simulink model "HybridControllerD3D3_Vconst"  (Simulink 7.9)
settings: Solver=FixedStepDiscrete  StartTime=0.0  StopTime=inf  RelTol=1e-3
PreLoadFcn:
  | initializeSimulation
values from neighbouring files (symbols this model uses):
  nAct = 8    [initializeSimulation.m]
  nDOF = 2    [initializeSimulation.m]
  nDout = 4    [initializeSimulation.m]
  node = completenodestruct(node)    [initializeSimulation.m]
undefined symbols (not defined in the file or in its folder): dofID, HybridCtrlParameters, vDOF, vDOFmax
libraries: xpclib x10, xpcsystranlib x4, simulink x4
CloseFcn:
  | rtwprivate ssgencode ModelCloseRequest scrnet_receiver
settings Model: Creator=Andreas Schellenberg  LastModifiedBy=Andreas  ExtModeArmWhenConnect=off  BufferReuse=off
settings DataIOCC: LimitDataPoints=off  SaveOutput=off  SignalLogging=off  SaveTime=off  SignalLoggingName=sigsOut
settings OptimizationCC: BlockReduction=off  OptimizeBlockIOStorage=off  BufferReuse=off  ExpressionFolding=off  FoldNonRolledExpr=off  LocalBlockOutputs=off  StateBitsets=on  DataBitsets=on  InitFltsAndDblsToZero=on  EfficientFloat2IntCast=on  SimCompilerOptimization=On
settings DebuggingCC: SaveWithParameterizedLinksMsg=none  CheckSSInitialOutputMsg=off  SolverPrmCheckMsg=none  FcnCallInpInsideContextMsg=Use local settings  StrictBusMsg=None
settings HardwareCC: ProdIntDivRoundTo=Zero  ProdEndianess=LittleEndian  ProdHWDeviceType=Generic->32-bit x86 compatible  TargetIntDivRoundTo=Zero  TargetEndianess=LittleEndian  TargetHWDeviceType=Intel->x86/Pentium
settings SFSimCC: SimCustomHeaderCode="#include \"PredictorCorrector.h\""  SimUserSources=PredictorCorrector.c  SimUserIncludeDirs=D:\PredictorCorrector\HybridSimToolbox  SimParseCustomCode=off
settings RTWCC: SystemTargetFile=xpctarget.tlc  TemplateMakefile=xpc_default_tmf  Description=xPC Target  ProcessScript=xpctarget_make_rtw_hook  CustomHeaderCode="#include \"PredictorCorrector.h\""  CustomInclude=D:\PredictorCorrector\HybridSimToolbox  CustomSource=PredictorCorrector.c  IncludeERTFirstTime=on  RTWCompilerOptimization=On
settings xpcTargetCC: TargetFcnLib=ansi_tfl_tmw.mat  CodeReplacementLibrary=XPC_BLAS  CodeExecutionProfiling=off  ParMdlRefBuildCompliant=on  ConcurrentExecutionCompliant=on  CombineSignalStateStructs=off  PortableWordSizes=off  GRTInterface=on  xPCTaskExecutionProfile=off  xPCRL32EventNumber=5000  RL32IRQSourceModifier=11  xPCIRQSourceBoard=Scramnet_SC150+  xPCLoadParamSetFile=off  xPCConcurrentTasks=off  xPCEnableSFAnimation=off

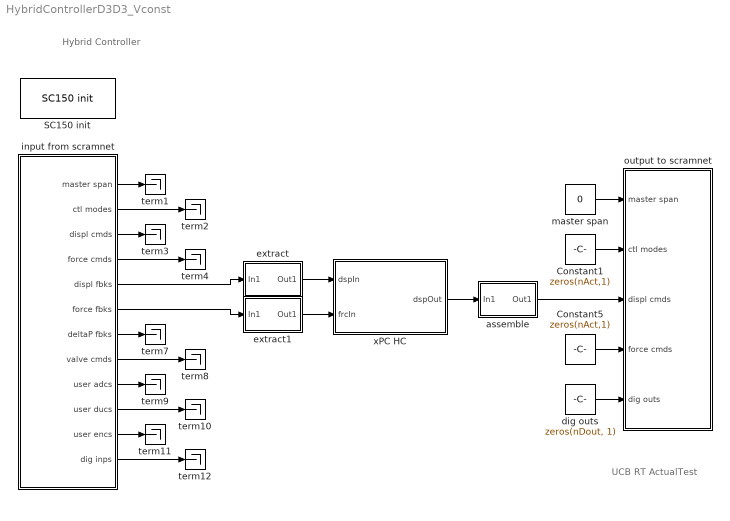
== system HybridControllerD3D3_Vconst ==
  note: Hybrid Controller
  note: UCB RT ActualTest
  Constant1 : Constant  Value=zeros(nAct,1)
  Constant5 : Constant  Value=zeros(nAct,1)
  SC150 init : xpcsystranlib/Shared Memory/SC150 init   node=node  pci=-1
  assemble : Subsystem  mask(to Actuators){id=[2 3], size=nAct}
      mask prompts: id "Index Vector: id"; size "Vector Size: size"
      mask help: To select to which actuator(s) the signals are going to
      mask Display: disp('Assemble')
  dig outs : Constant  Value=zeros(nDout, 1)  OutDataTypeStr=uint32
  extract : Subsystem  mask(from Actuators){id=[2 3], size=nAct}
      mask prompts: id "Index Vector: id"; size "Vector Size: size"
      mask help: To select from which actuator(s) the signals are coming from
      mask Display: disp('Extract')
  extract1 : Subsystem  mask(from Actuators){id=[2 3], size=nAct}
      mask prompts: id "Index Vector: id"; size "Vector Size: size"
      mask help: To select from which actuator(s) the signals are coming from
      mask Display: disp('Extract')
  input from scramnet : Subsystem
  master span : Constant  Value=0
  output to scramnet : Subsystem
  term{1..4,7..12} (10 alike) : Terminator
  xPC HC : Subsystem  mask(Hybrid Controller: D3/D3){nDOF=nDOF, dtInt=HybridCtrlParameters.dtInt, dtSim=HybridCtrlParameters.dtSim, dtCon=HybridCtrlParameters.dtCon, N=HybridCtrlParameters.N, iDelay=HybridCtrlParameters.iDelay}
      mask prompts: nDOF "Number of DOF: nDOF"; dtInt "Integration time step: dtInt"; dtSim "Simulation time step: dtSim"; dtCon "Controller time step: dtCon"; N "Maximum number of substeps: N"; iDelay "Number of delay steps: iDelay"
      mask help: Hybrid Controller using C0-continuous cubic Lagrange interpolation for prediction and correction
      mask Display: disp('xPC Target\nHybrid Controller\n(D3/D3 Vconst)')
  wires:
  input from scramnet/10(user ducs) -> term10/1
  input from scramnet/12(dig inps) -> term12/1
  input from scramnet/2(ctl modes) -> term2/1
  input from scramnet/4(force cmds) -> term4/1
  input from scramnet/8(valve cmds) -> term8/1
  input from scramnet/1(master span) -> term1/1
  input from scramnet/7(deltaP fbks) -> term7/1
  input from scramnet/9(user adcs) -> term9/1
  input from scramnet/11(user encs) -> term11/1
  master span/1 -> output to scramnet/1(master span)
  Constant5/1 -> output to scramnet/4(force cmds)
  Constant1/1 -> output to scramnet/2(ctl modes)
  input from scramnet/3(displ cmds) -> term3/1
  input from scramnet/5(displ fbks) -> extract/1(In1)
  dig outs/1 -> output to scramnet/5(dig outs)
  extract/1(Out1) -> xPC HC/1(dspIn)
  xPC HC/1(dspOut) -> assemble/1(In1)
  assemble/1(Out1) -> output to scramnet/3(displ cmds)
  input from scramnet/6(force fbks) -> extract1/1(In1)
  extract1/1(Out1) -> xPC HC/2(frcIn)

== system HybridControllerD3D3_Vconst/assemble ==
  In1 : Inport
  Assignment : Assignment  OutputInitialize=Specify size for each dimension in table  IndexOptions=Index vector (port)  Indices=1  OutputSizes=size
  Constant : Constant  Value=id
  Out1 : Outport
  wires:
  Constant/1 -> Assignment/2
  Assignment/1 -> Out1/1
  In1/1 -> Assignment/1

== system HybridControllerD3D3_Vconst/extract ==
  In1 : Inport
  Selector : Selector  InputPortWidth=size  IndexOptions=Index vector (dialog)  Indices=id  OutputSizes=1
  Out1 : Outport
  wires:
  Selector/1 -> Out1/1
  In1/1 -> Selector/1

== system HybridControllerD3D3_Vconst/extract1 ==
  In1 : Inport
  Selector : Selector  InputPortWidth=size  IndexOptions=Index vector (dialog)  Indices=id  OutputSizes=1
  Out1 : Outport
  wires:
  Selector/1 -> Out1/1
  In1/1 -> Selector/1

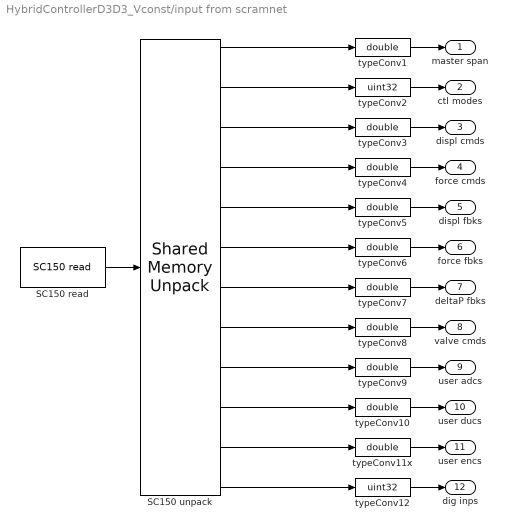
== system HybridControllerD3D3_Vconst/input from scramnet ==
  SC150 read : xpcsystranlib/Shared Memory/SC150 read   partition=node.Partitions(12:23)  errorport=off  ts=samplePeriod  pci=-1
  SC150 unpack : xpclib/Shared Memory/Shared Memory Unpack   partition=node.Partitions(12:23)
  typeConv{1,3..10} (9 alike) : DataTypeConversion  OutDataTypeStr=double  SaturateOnIntegerOverflow=on  RndMeth=Zero
  typeConv11x : DataTypeConversion  OutDataTypeStr=double  SaturateOnIntegerOverflow=on  RndMeth=Zero
  typeConv12 : DataTypeConversion  OutDataTypeStr=uint32  SaturateOnIntegerOverflow=on  RndMeth=Zero
  typeConv2 : DataTypeConversion  OutDataTypeStr=uint32  SaturateOnIntegerOverflow=on  RndMeth=Zero
  master span : Outport
  ctl modes : Outport  Port=2
  displ cmds : Outport  Port=3
  force cmds : Outport  Port=4
  displ fbks : Outport  Port=5
  force fbks : Outport  Port=6
  deltaP fbks : Outport  Port=7
  valve cmds : Outport  Port=8
  user adcs : Outport  Port=9
  user ducs : Outport  Port=10
  user encs : Outport  Port=11
  dig inps : Outport  Port=12
  wires:
  typeConv11x/1 -> user encs/1
  typeConv10/1 -> user ducs/1
  typeConv12/1 -> dig inps/1
  typeConv9/1 -> user adcs/1
  typeConv8/1 -> valve cmds/1
  typeConv7/1 -> deltaP fbks/1
  typeConv6/1 -> force fbks/1
  typeConv5/1 -> displ fbks/1
  typeConv4/1 -> force cmds/1
  typeConv3/1 -> displ cmds/1
  typeConv1/1 -> master span/1
  SC150 read/1 -> SC150 unpack/1
  typeConv2/1 -> ctl modes/1
  SC150 unpack/1 -> typeConv1/1
  SC150 unpack/2 -> typeConv2/1
  SC150 unpack/3 -> typeConv3/1
  SC150 unpack/4 -> typeConv4/1
  SC150 unpack/5 -> typeConv5/1
  SC150 unpack/6 -> typeConv6/1
  SC150 unpack/7 -> typeConv7/1
  SC150 unpack/8 -> typeConv8/1
  SC150 unpack/9 -> typeConv9/1
  SC150 unpack/10 -> typeConv10/1
  SC150 unpack/11 -> typeConv11x/1
  SC150 unpack/12 -> typeConv12/1

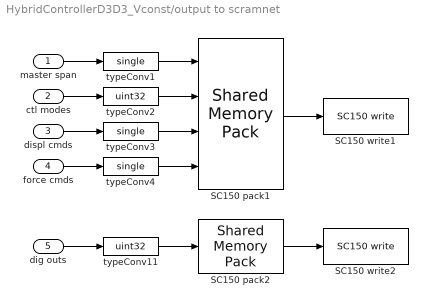
== system HybridControllerD3D3_Vconst/output to scramnet ==
  master span : Inport
  ctl modes : Inport  Port=2
  displ cmds : Inport  Port=3
  force cmds : Inport  Port=4
  dig outs : Inport  Port=5
  SC150 pack1 : xpclib/Shared Memory/Shared Memory Pack   partition=node.Partitions(1:4)
  SC150 pack2 : xpclib/Shared Memory/Shared Memory Pack   partition=node.Partitions(11)
  SC150 write1 : xpcsystranlib/Shared Memory/SC150 write   partition=node.Partitions(1:4)  errorport=off  ts=samplePeriod  pci=-1
  SC150 write2 : xpcsystranlib/Shared Memory/SC150 write   partition=node.Partitions(11)  errorport=off  ts=samplePeriod  pci=-1
  typeConv1 : DataTypeConversion  OutDataTypeStr=single  SaturateOnIntegerOverflow=on  RndMeth=Zero
  typeConv11 : DataTypeConversion  OutDataTypeStr=uint32  SaturateOnIntegerOverflow=on  RndMeth=Zero
  typeConv2 : DataTypeConversion  OutDataTypeStr=uint32  SaturateOnIntegerOverflow=on  RndMeth=Zero
  typeConv3 : DataTypeConversion  OutDataTypeStr=single  SaturateOnIntegerOverflow=on  RndMeth=Zero
  typeConv4 : DataTypeConversion  OutDataTypeStr=single  SaturateOnIntegerOverflow=on  RndMeth=Zero
  wires:
  dig outs/1 -> typeConv11/1
  force cmds/1 -> typeConv4/1
  master span/1 -> typeConv1/1
  SC150 pack1/1 -> SC150 write1/1
  displ cmds/1 -> typeConv3/1
  ctl modes/1 -> typeConv2/1
  typeConv1/1 -> SC150 pack1/1
  typeConv2/1 -> SC150 pack1/2
  typeConv3/1 -> SC150 pack1/3
  typeConv4/1 -> SC150 pack1/4
  SC150 pack2/1 -> SC150 write2/1
  typeConv11/1 -> SC150 pack2/1

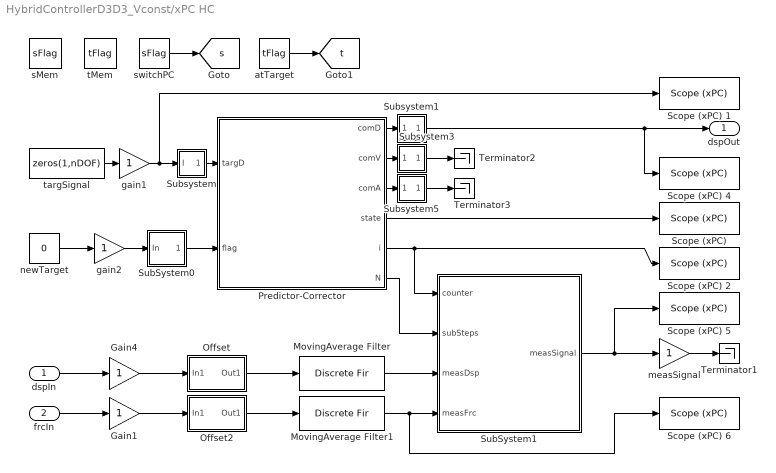
== system HybridControllerD3D3_Vconst/xPC HC ==
  dspIn : Inport
  frcIn : Inport  Port=2
  Gain1 : Gain  SaturateOnIntegerOverflow=on  OutDataTypeStr=Inherit: Same as input  ParamDataTypeStr=Inherit: Same as input
  Gain4 : Gain  SaturateOnIntegerOverflow=on  OutDataTypeStr=Inherit: Same as input  ParamDataTypeStr=Inherit: Same as input
  MovingAverage Filter : DiscreteFir  Coefficients=1/numSample*ones(1,numSample)  mask(Moving Average Filter){numSample=1}
      mask prompts: numSample "Number of Samples: numSample"
      mask help:
      | Moving average filter by using discrete FIR filter.
      | Set numSample = 1 for no filtering.
      mask Display: fprintf('MovingAverage\nFilter')
  MovingAverage Filter1 : DiscreteFir  Coefficients=1/numSample*ones(1,numSample)  mask(Moving Average Filter){numSample=1}
      mask prompts: numSample "Number of Samples: numSample"
      mask help:
      | Moving average filter by using discrete FIR filter.
      | Set numSample = 1 for no filtering.
      mask Display: fprintf('MovingAverage\nFilter')
  Offset : Subsystem  mask(Signal Offset){nS=nDOF, nOffset=-1, dt=dtCon}
      mask prompts: nS "Number of Signals: nS"; nOffset "Number of samples to initialize offset: nOffset"; dt "Sample time: dt"
      mask help:
      | Offset signal by average of signal over initial number of samples.
      | Set nOffset = -1 for no signal offset.
      mask Display: fprintf('Signal\nOffset')
  Offset2 : Subsystem  mask(Signal Offset){nS=nDOF, nOffset=-1, dt=dtCon}
      mask prompts: nS "Number of Signals: nS"; nOffset "Number of samples to initialize offset: nOffset"; dt "Sample time: dt"
      mask help:
      | Offset signal by average of signal over initial number of samples.
      | Set nOffset = -1 for no signal offset.
      mask Display: fprintf('Signal\nOffset')
  Predictor-Corrector : Stateflow chart  TreatAsAtomicUnit=on
  "Scope (xPC) " : xpclib/Misc./Scope (xPC)   scopeno=8  scopetype=File  autostart=on  viewmode=Graphical redraw  formatstr='%15.6f'  grid=on  ylimits=[0,3]  nosamples=4096  noprepostsamples=0  interleave=1  triggermode=FreeRun  triggersignal=1  triggerlevel=0.0  triggerslope=Either  triggerscope=1  triggersample=0  filename=state1.dat  mode=Lazy  writesize=512  autorestart=on  dynamicfilemode=off  maxwritefilesize=512*1024^2
  Scope (xPC) 1 : xpclib/Misc./Scope (xPC)   scopeno=4  scopetype=File  autostart=on  viewmode=Numerical  formatstr='%15.6f'  grid=on  ylimits=[-4,4]  nosamples=4096  noprepostsamples=0  interleave=1  triggermode=FreeRun  triggersignal=1  triggerlevel=0.0  triggerslope=Either  triggerscope=1  triggersample=0  filename=targDsp1.dat  mode=Lazy  writesize=512  autorestart=on  dynamicfilemode=off  maxwritefilesize=512*1024^2
  Scope (xPC) 2 : xpclib/Misc./Scope (xPC)   scopeno=1  scopetype=File  autostart=on  viewmode=Numerical  formatstr='%15.6f'  grid=on  ylimits=[0,3]  nosamples=4096  noprepostsamples=0  interleave=1  triggermode=FreeRun  triggersignal=1  triggerlevel=0.0  triggerslope=Either  triggerscope=1  triggersample=0  filename=count1.dat  mode=Lazy  writesize=512  autorestart=on  dynamicfilemode=off  maxwritefilesize=512*1024^2
  Scope (xPC) 4 : xpclib/Misc./Scope (xPC)   scopeno=5  scopetype=File  autostart=on  viewmode=Numerical  formatstr='%15.6f'  grid=on  ylimits=[-4,4]  nosamples=4096  noprepostsamples=0  interleave=1  triggermode=FreeRun  triggersignal=1  triggerlevel=0.0  triggerslope=Either  triggerscope=1  triggersample=0  filename=commDsp1.dat  mode=Lazy  writesize=512  autorestart=on  dynamicfilemode=off  maxwritefilesize=512*1024^2
  Scope (xPC) 5 : xpclib/Misc./Scope (xPC)   scopeno=2  scopetype=File  autostart=on  viewmode=Numerical  formatstr='%15.6f'  grid=on  ylimits=[-4,4]  nosamples=4096  noprepostsamples=0  interleave=1  triggermode=FreeRun  triggersignal=1  triggerlevel=0.0  triggerslope=Either  triggerscope=1  triggersample=0  filename=measDsp1.dat  mode=Lazy  writesize=512  autorestart=on  dynamicfilemode=off  maxwritefilesize=512*1024^2
  Scope (xPC) 6 : xpclib/Misc./Scope (xPC)   scopeno=3  scopetype=File  autostart=on  viewmode=Numerical  formatstr='%15.6f'  grid=on  ylimits=[0,3]  nosamples=4096  noprepostsamples=0  interleave=1  triggermode=FreeRun  triggersignal=1  triggerlevel=0.0  triggerslope=Either  triggerscope=1  triggersample=0  filename=measFrc1.dat  mode=Lazy  writesize=512  autorestart=on  dynamicfilemode=off  maxwritefilesize=512*1024^2
  SubSystem0 : Subsystem
  SubSystem1 : Subsystem
  Subsystem : Subsystem
      mask Display: disp('I/O')
  Subsystem1 : Subsystem
      mask Display: disp('I/O')
  Subsystem3 : Subsystem
      mask Display: disp('I/O')
  Subsystem5 : Subsystem
      mask Display: disp('I/O')
  Terminator1 : Terminator
  Terminator2 : Terminator
  Terminator3 : Terminator
  atTarget : DataStoreRead  DataStoreName=tFlag  SampleTime=dtCon
  gain1 : Gain
  gain2 : Gain
  measSignal : Gain
  newTarget : Constant  Value=0  SampleTime=dtCon
  sMem : DataStoreMemory  DataStoreName=sFlag  OutDataTypeStr=double
  switchPC : DataStoreRead  DataStoreName=sFlag  SampleTime=dtCon
  tMem : DataStoreMemory  DataStoreName=tFlag  OutDataTypeStr=double
  targSignal : Constant  Value=zeros(1,nDOF)  SampleTime=dtCon
  dspOut : Outport
  tag scope: s=global, t=global
  wires:
  frcIn/1 -> Gain1/1
  measSignal/1 -> Terminator1/1
  dspIn/1 -> Gain4/1
  SubSystem1/1(measSignal) -> measSignal/1, Scope (xPC) 5/1
  Predictor-Corrector/5(i) -> Scope (xPC) 2/1, SubSystem1/1(counter)
  Predictor-Corrector/4(state) -> "Scope (xPC) "/1
  Offset/1(Out1) -> MovingAverage Filter/1
  SubSystem0/1(Out) -> Predictor-Corrector/2(flag)
  newTarget/1 -> gain2/1
  gain2/1 -> SubSystem0/1(In)
  switchPC/1 -> [s]
  atTarget/1 -> [t]
  targSignal/1 -> gain1/1
  gain1/1 -> Scope (xPC) 1/1, Subsystem/1(I)
  Subsystem1/1(Out) -> dspOut/1, Scope (xPC) 4/1
  Subsystem/1(O) -> Predictor-Corrector/1(targD)
  MovingAverage Filter/1 -> SubSystem1/3(measDsp)
  MovingAverage Filter1/1 -> Scope (xPC) 6/1, SubSystem1/4(measFrc)
  Predictor-Corrector/1(comD) -> Subsystem1/1(In)
  Predictor-Corrector/2(comV) -> Subsystem3/1(In)
  Predictor-Corrector/3(comA) -> Subsystem5/1(In)
  Subsystem3/1(Out) -> Terminator2/1
  Subsystem5/1(Out) -> Terminator3/1
  Gain4/1 -> Offset/1(In1)
  Gain1/1 -> Offset2/1(In1)
  Offset2/1(Out1) -> MovingAverage Filter1/1
  Predictor-Corrector/6(N) -> SubSystem1/2(subSteps)

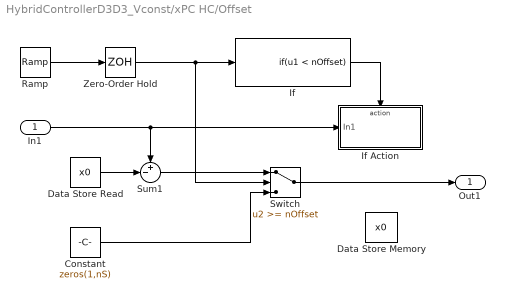
== system HybridControllerD3D3_Vconst/xPC HC/Offset ==
  In1 : Inport
  Constant : Constant  Value=zeros(1,nS)
  Data Store Memory : DataStoreMemory  DataStoreName=x0  InitialValue=zeros(1,nS)  OutDataTypeStr=double
  Data Store Read : DataStoreRead  DataStoreName=x0  SampleTime=dt
  If : If  IfExpression=u1 < nOffset  ShowElse=off
  If Action : Subsystem  TreatAsAtomicUnit=on
  Ramp : simulink/Sources/Ramp  slope=1/dt  start=0  X0=0
  Sum1 : Sum  Inputs=+-|  SaturateOnIntegerOverflow=on  InputSameDT=on  OutDataTypeStr=Inherit: Same as first input
  Switch : Switch  Threshold=nOffset  SaturateOnIntegerOverflow=on  InputSameDT=on
  Zero-Order Hold : ZeroOrderHold  SampleTime=dt
  Out1 : Outport
  wires:
  Switch/1 -> Out1/1
  Sum1/1 -> Switch/1
  Data Store Read/1 -> Sum1/2
  In1/1 -> If Action/1(In1), Sum1/1
  Constant/1 -> Switch/3
  Zero-Order Hold/1 -> Switch/2, If/1
  If/1 -> If Action/Action
  Ramp/1 -> Zero-Order Hold/1

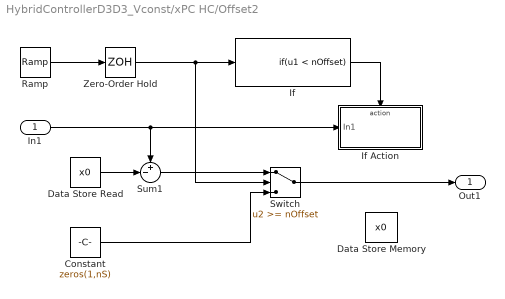
== system HybridControllerD3D3_Vconst/xPC HC/Offset2 ==
  In1 : Inport
  Constant : Constant  Value=zeros(1,nS)
  Data Store Memory : DataStoreMemory  DataStoreName=x0  InitialValue=zeros(1,nS)  OutDataTypeStr=double
  Data Store Read : DataStoreRead  DataStoreName=x0  SampleTime=dt
  If : If  IfExpression=u1 < nOffset  ShowElse=off
  If Action : Subsystem  TreatAsAtomicUnit=on
  Ramp : simulink/Sources/Ramp  slope=1/dt  start=0  X0=0
  Sum1 : Sum  Inputs=+-|  SaturateOnIntegerOverflow=on  InputSameDT=on  OutDataTypeStr=Inherit: Same as first input
  Switch : Switch  Threshold=nOffset  SaturateOnIntegerOverflow=on  InputSameDT=on
  Zero-Order Hold : ZeroOrderHold  SampleTime=dt
  Out1 : Outport
  wires:
  Ramp/1 -> Zero-Order Hold/1
  If/1 -> If Action/Action
  Zero-Order Hold/1 -> If/1, Switch/2
  Constant/1 -> Switch/3
  In1/1 -> Sum1/1, If Action/1(In1)
  Data Store Read/1 -> Sum1/2
  Sum1/1 -> Switch/1
  Switch/1 -> Out1/1

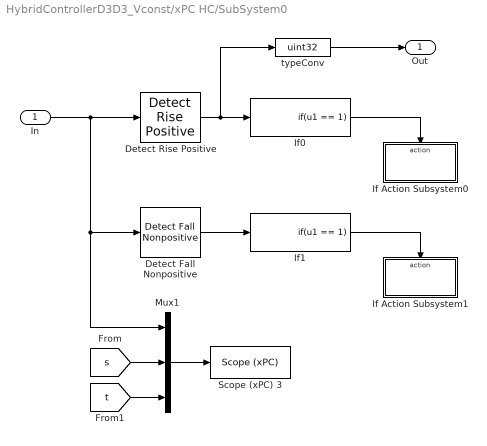
== system HybridControllerD3D3_Vconst/xPC HC/SubSystem0 ==
  In : Inport
  Detect Fall Nonpositive : simulink/Logic and Bit Operations/Detect Fall Nonpositive  vinit=0  InputProcessing=Inherited  OutDataTypeStr=uint8
  Detect Rise Positive : simulink/Logic and Bit Operations/Detect Rise Positive  vinit=0  InputProcessing=Inherited  OutDataTypeStr=uint8
  If Action Subsystem0 : Subsystem  TreatAsAtomicUnit=on
  If Action Subsystem1 : Subsystem  TreatAsAtomicUnit=on
  If0 : If  IfExpression=u1 == 1  ShowElse=off
  If1 : If  IfExpression=u1 == 1  ShowElse=off
  Mux1 : Mux  Inputs=3
  Scope (xPC) 3 : xpclib/Misc./Scope (xPC)   scopeno=6  scopetype=File  autostart=on  viewmode=Numerical  formatstr='%15.6f'  grid=on  ylimits=[0,3]  nosamples=4096  noprepostsamples=0  interleave=1  triggermode=FreeRun  triggersignal=1  triggerlevel=0.0  triggerslope=Either  triggerscope=1  triggersample=0  filename=flag1.dat  mode=Lazy  writesize=512  autorestart=on  dynamicfilemode=off  maxwritefilesize=512*1024^2
  typeConv : DataTypeConversion  OutDataTypeStr=uint32  SaturateOnIntegerOverflow=on  RndMeth=Zero
  Out : Outport
  wires:
  In/1 -> Detect Rise Positive/1, Detect Fall Nonpositive/1, Mux1/1
  Detect Rise Positive/1 -> If0/1, typeConv/1
  Detect Fall Nonpositive/1 -> If1/1
  If1/1 -> If Action Subsystem1/Action
  If0/1 -> If Action Subsystem0/Action
  typeConv/1 -> Out/1
  Mux1/1 -> Scope (xPC) 3/1
  [s] -> Mux1/2
  [t] -> Mux1/3

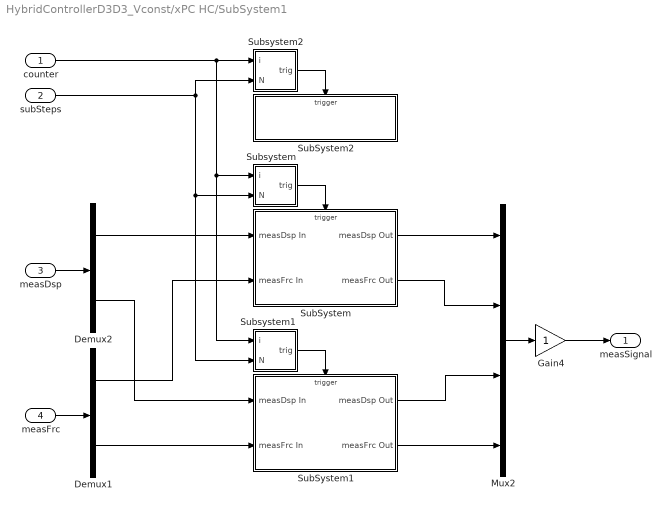
== system HybridControllerD3D3_Vconst/xPC HC/SubSystem1 ==
  counter : Inport
  subSteps : Inport  Port=2
  measDsp : Inport  Port=3
  measFrc : Inport  Port=4
  Demux1 : Demux  Outputs=2
  Demux2 : Demux  Outputs=2
  Gain4 : Gain  SaturateOnIntegerOverflow=on  OutDataTypeStr=Inherit: Same as input  ParamDataTypeStr=Inherit: Same as input
  Mux2 : Mux
  SubSystem : Subsystem  TreatAsAtomicUnit=on
  SubSystem1 : Subsystem  TreatAsAtomicUnit=on
  SubSystem2 : Subsystem  TreatAsAtomicUnit=on
  Subsystem : Subsystem
  Subsystem1 : Subsystem
  Subsystem2 : Subsystem
  measSignal : Outport
  wires:
  Subsystem/1(trig) -> SubSystem/Trigger
  Subsystem1/1(trig) -> SubSystem1/Trigger
  Subsystem2/1(trig) -> SubSystem2/Trigger
  Mux2/1 -> Gain4/1
  SubSystem/1(measDsp Out) -> Mux2/1
  counter/1 -> Subsystem/1(i), Subsystem1/1(i), Subsystem2/1(i)
  Gain4/1 -> measSignal/1
  SubSystem/2(measFrc Out) -> Mux2/2
  SubSystem1/1(measDsp Out) -> Mux2/3
  SubSystem1/2(measFrc Out) -> Mux2/4
  measDsp/1 -> Demux2/1
  measFrc/1 -> Demux1/1
  Demux2/1 -> SubSystem/1(measDsp In)
  Demux2/2 -> SubSystem1/1(measDsp In)
  Demux1/1 -> SubSystem/2(measFrc In)
  Demux1/2 -> SubSystem1/2(measFrc In)
  subSteps/1 -> Subsystem2/2(N), Subsystem/2(N), Subsystem1/2(N)

== system HybridControllerD3D3_Vconst/xPC HC/Subsystem ==
  I : Inport  PortDimensions=nAct
  Dummy Aug : Mux  Inputs=[nAct 1]
  Dummy Zero : Constant  Value=0  OutDataTypeStr=double  SampleTime=dtCon
  O : Outport  PortDimensions=nAct+1
  wires:
  Dummy Zero/1 -> Dummy Aug/2
  I/1 -> Dummy Aug/1
  Dummy Aug/1 -> O/1

== system HybridControllerD3D3_Vconst/xPC HC/Subsystem1 ==
  In : Inport  PortDimensions=nAct+1
  Dummy Trn : Demux  Outputs=[nAct 1]
  Terminator3 : Terminator
  Out : Outport  PortDimensions=nAct
  wires:
  Dummy Trn/2 -> Terminator3/1
  Dummy Trn/1 -> Out/1
  In/1 -> Dummy Trn/1

== system HybridControllerD3D3_Vconst/xPC HC/Subsystem3 ==
  In : Inport  PortDimensions=nAct+1
  Dummy Trn : Demux  Outputs=[nAct 1]
  Terminator3 : Terminator
  Out : Outport  PortDimensions=nAct
  wires:
  Dummy Trn/2 -> Terminator3/1
  Dummy Trn/1 -> Out/1
  In/1 -> Dummy Trn/1

== system HybridControllerD3D3_Vconst/xPC HC/Subsystem5 ==
  In : Inport  PortDimensions=nAct+1
  Dummy Trn : Demux  Outputs=[nAct 1]
  Terminator3 : Terminator
  Out : Outport  PortDimensions=nAct
  wires:
  Dummy Trn/2 -> Terminator3/1
  Dummy Trn/1 -> Out/1
  In/1 -> Dummy Trn/1

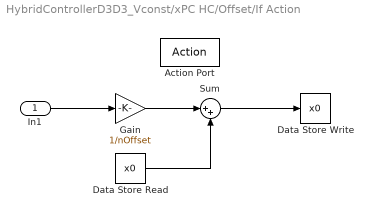
== system HybridControllerD3D3_Vconst/xPC HC/Offset/If Action ==
  In1 : Inport
  Action Port : ActionPort  PropagateVarSize=During execution
  Data Store Read : DataStoreRead  DataStoreName=x0  SampleTime=dt
  Data Store Write : DataStoreWrite  DataStoreName=x0
  Gain : Gain  Gain=1/nOffset  SaturateOnIntegerOverflow=on  OutDataTypeStr=Inherit: Same as input  ParamDataTypeStr=Inherit: Same as input
  Sum : Sum  Inputs=|++  SaturateOnIntegerOverflow=on  InputSameDT=on  OutDataTypeStr=Inherit: Same as first input
  wires:
  Data Store Read/1 -> Sum/2
  Sum/1 -> Data Store Write/1
  Gain/1 -> Sum/1
  In1/1 -> Gain/1

== system HybridControllerD3D3_Vconst/xPC HC/Offset2/If Action ==
  In1 : Inport
  Action Port : ActionPort  PropagateVarSize=During execution
  Data Store Read : DataStoreRead  DataStoreName=x0  SampleTime=dt
  Data Store Write : DataStoreWrite  DataStoreName=x0
  Gain : Gain  Gain=1/nOffset  SaturateOnIntegerOverflow=on  OutDataTypeStr=Inherit: Same as input  ParamDataTypeStr=Inherit: Same as input
  Sum : Sum  Inputs=|++  SaturateOnIntegerOverflow=on  InputSameDT=on  OutDataTypeStr=Inherit: Same as first input
  wires:
  In1/1 -> Gain/1
  Gain/1 -> Sum/1
  Sum/1 -> Data Store Write/1
  Data Store Read/1 -> Sum/2

== system HybridControllerD3D3_Vconst/xPC HC/SubSystem0/If Action Subsystem0 ==
  Action Port : ActionPort  PropagateVarSize=During execution
  Data Store Write0 : DataStoreWrite  DataStoreName=sFlag
  Data Store Write1 : DataStoreWrite  DataStoreName=tFlag
  atTargetFlag : Constant  Value=0  SampleTime=dtCon
  switchFlag : Constant  SampleTime=dtCon
  wires:
  atTargetFlag/1 -> Data Store Write1/1
  switchFlag/1 -> Data Store Write0/1

== system HybridControllerD3D3_Vconst/xPC HC/SubSystem0/If Action Subsystem1 ==
  Action Port : ActionPort  PropagateVarSize=During execution
  Data Store Write0 : DataStoreWrite  DataStoreName=sFlag
  switchFlag : Constant  Value=0  SampleTime=dtCon
  wires:
  switchFlag/1 -> Data Store Write0/1

== system HybridControllerD3D3_Vconst/xPC HC/SubSystem1/SubSystem ==
  measDsp In : Inport
  measFrc In : Inport  Port=2
  Trigger : TriggerPort
  measDsp Out : Outport  InitialOutput=[0]
  measFrc Out : Outport  Port=2  InitialOutput=[0]
  wires:
  measFrc In/1 -> measFrc Out/1
  measDsp In/1 -> measDsp Out/1

== system HybridControllerD3D3_Vconst/xPC HC/SubSystem1/SubSystem1 ==
  measDsp In : Inport
  measFrc In : Inport  Port=2
  Trigger : TriggerPort
  measDsp Out : Outport  InitialOutput=[0]
  measFrc Out : Outport  Port=2  InitialOutput=[0]
  wires:
  measFrc In/1 -> measFrc Out/1
  measDsp In/1 -> measDsp Out/1

== system HybridControllerD3D3_Vconst/xPC HC/SubSystem1/SubSystem2 ==
  Trigger : TriggerPort
  Data Store Write : DataStoreWrite  DataStoreName=tFlag
  atTargetFlag : Constant  OutDataTypeStr=uint32  SampleTime=-1
  wires:
  atTargetFlag/1 -> Data Store Write/1

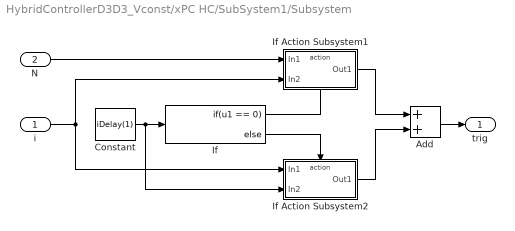
== system HybridControllerD3D3_Vconst/xPC HC/SubSystem1/Subsystem ==
  i : Inport
  N : Inport  Port=2
  Add : Sum
  Constant : Constant  Value=iDelay(1)
  If : If  IfExpression=u1 == 0
  If Action Subsystem1 : Subsystem  TreatAsAtomicUnit=on
  If Action Subsystem2 : Subsystem  TreatAsAtomicUnit=on
  trig : Outport
  wires:
  Constant/1 -> If/1, If Action Subsystem2/2(In2)
  If/1 -> If Action Subsystem1/Action
  If/2 -> If Action Subsystem2/Action
  If Action Subsystem1/1(Out1) -> Add/1
  If Action Subsystem2/1(Out1) -> Add/2
  Add/1 -> trig/1
  i/1 -> If Action Subsystem1/2(In2), If Action Subsystem2/1(In1)
  N/1 -> If Action Subsystem1/1(In1)

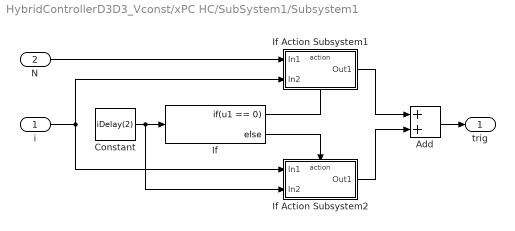
== system HybridControllerD3D3_Vconst/xPC HC/SubSystem1/Subsystem1 ==
  i : Inport
  N : Inport  Port=2
  Add : Sum
  Constant : Constant  Value=iDelay(2)
  If : If  IfExpression=u1 == 0
  If Action Subsystem1 : Subsystem  TreatAsAtomicUnit=on
  If Action Subsystem2 : Subsystem  TreatAsAtomicUnit=on
  trig : Outport
  wires:
  Constant/1 -> If/1, If Action Subsystem2/2(In2)
  If/1 -> If Action Subsystem1/Action
  If/2 -> If Action Subsystem2/Action
  If Action Subsystem1/1(Out1) -> Add/1
  If Action Subsystem2/1(Out1) -> Add/2
  Add/1 -> trig/1
  i/1 -> If Action Subsystem1/2(In2), If Action Subsystem2/1(In1)
  N/1 -> If Action Subsystem1/1(In1)

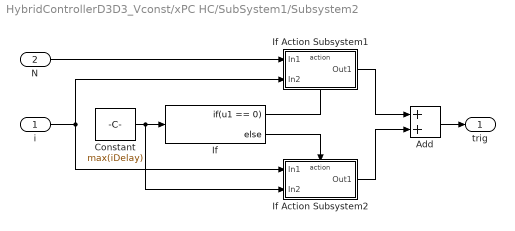
== system HybridControllerD3D3_Vconst/xPC HC/SubSystem1/Subsystem2 ==
  i : Inport
  N : Inport  Port=2
  Add : Sum
  Constant : Constant  Value=max(iDelay)
  If : If  IfExpression=u1 == 0
  If Action Subsystem1 : Subsystem  TreatAsAtomicUnit=on
  If Action Subsystem2 : Subsystem  TreatAsAtomicUnit=on
  trig : Outport
  wires:
  Constant/1 -> If/1, If Action Subsystem2/2(In2)
  If/1 -> If Action Subsystem1/Action
  If/2 -> If Action Subsystem2/Action
  If Action Subsystem1/1(Out1) -> Add/1
  If Action Subsystem2/1(Out1) -> Add/2
  Add/1 -> trig/1
  i/1 -> If Action Subsystem1/2(In2), If Action Subsystem2/1(In1)
  N/1 -> If Action Subsystem1/1(In1)

== system HybridControllerD3D3_Vconst/xPC HC/SubSystem1/Subsystem/If Action Subsystem1 ==
  In1 : Inport
  In2 : Inport  Port=2
  Action Port : ActionPort
  Relational Operator : RelationalOperator  Operator===  OutDataTypeStr=boolean
  Out1 : Outport
  wires:
  Relational Operator/1 -> Out1/1
  In1/1 -> Relational Operator/1
  In2/1 -> Relational Operator/2

== system HybridControllerD3D3_Vconst/xPC HC/SubSystem1/Subsystem/If Action Subsystem2 ==
  In1 : Inport
  In2 : Inport  Port=2
  Action Port : ActionPort
  Relational Operator : RelationalOperator  Operator===  OutDataTypeStr=boolean
  Out1 : Outport
  wires:
  Relational Operator/1 -> Out1/1
  In1/1 -> Relational Operator/1
  In2/1 -> Relational Operator/2

== system HybridControllerD3D3_Vconst/xPC HC/SubSystem1/Subsystem1/If Action Subsystem1 ==
  In1 : Inport
  In2 : Inport  Port=2
  Action Port : ActionPort
  Relational Operator : RelationalOperator  Operator===  OutDataTypeStr=boolean
  Out1 : Outport
  wires:
  Relational Operator/1 -> Out1/1
  In1/1 -> Relational Operator/1
  In2/1 -> Relational Operator/2

== system HybridControllerD3D3_Vconst/xPC HC/SubSystem1/Subsystem1/If Action Subsystem2 ==
  In1 : Inport
  In2 : Inport  Port=2
  Action Port : ActionPort
  Relational Operator : RelationalOperator  Operator===  OutDataTypeStr=boolean
  Out1 : Outport
  wires:
  Relational Operator/1 -> Out1/1
  In1/1 -> Relational Operator/1
  In2/1 -> Relational Operator/2

== system HybridControllerD3D3_Vconst/xPC HC/SubSystem1/Subsystem2/If Action Subsystem1 ==
  In1 : Inport
  In2 : Inport  Port=2
  Action Port : ActionPort
  Relational Operator : RelationalOperator  Operator===  OutDataTypeStr=boolean
  Out1 : Outport
  wires:
  Relational Operator/1 -> Out1/1
  In1/1 -> Relational Operator/1
  In2/1 -> Relational Operator/2

== system HybridControllerD3D3_Vconst/xPC HC/SubSystem1/Subsystem2/If Action Subsystem2 ==
  In1 : Inport
  In2 : Inport  Port=2
  Action Port : ActionPort
  Relational Operator : RelationalOperator  Operator===  OutDataTypeStr=boolean
  Out1 : Outport
  wires:
  Relational Operator/1 -> Out1/1
  In1/1 -> Relational Operator/1
  In2/1 -> Relational Operator/2

== stateflow chart xPC HC/Predictor-Corrector ==
  state HybridController [parallel]
    settings: executionOrder=1
    state Predict
      en: state = 1;
      en: setCurSig(comD,i/N);
      en: diSD = 1;
      en: i = 1; iSD = 0;
      en: N = getNumSubSteps(vDOF,dofID,
      vDOFmax,ceil(max(iDelay)/0.6));
      en: predictD3(comD,i/N);
      en: predictV2(comV,i/N); predictA2(comA,i/N);
      du: i++;
      du: predictD3(comD,i/N);
      du: predictV2(comV,i/N); predictA2(comA,i/N);
    state Initialize
      en: i = 1; iSD = 0;
      en: diSD = 1;
      en: initData(nDOF,dtCon,dtSim,dtInt);
      en: zeroSig(comD);
      en: zeroSig(comV);
      en: zeroSig(comA);
    state AutoSlowDown
      en: state = 2;
      en: diSD = 4-i/(0.2*N);
      en: i += diSD; iSD = i;
      en: predictD3(comD,i/N);
      en: predictV2(comV,i/N); predictA2(comA,i/N);
      du: diSD = 4-i/(0.2*N);
      du: i += diSD; iSD = i;
      du: predictD3(comD,i/N);
      du: predictV2(comV,i/N); predictA2(comA,i/N);
    state Correct
      en: state = 0;
      en: setCurSig(comD,i/N);
      en: targLocal = targD; setNewSig(targLocal);
      en: di = min(max(diSD+1/(0.2*N)*(i-iSD),0.001),1.0);
      en: i = min(i+di,N);
      en: correctD3(comD,i/N);
      en: correctV2(comV,i/N); correctA2(comA,i/N);
      du: di = min(max(diSD+1/(0.2*N)*(i-iSD),0.001),1.0);
      du: i = min(i+di,N);
      du: correctD3(comD,i/N);
      du: correctV2(comV,i/N); correctA2(comA,i/N);
    Correct -> Predict [order 1] : [i>=N && flag!=1]
    (default) -> Initialize
    Initialize -> Correct : [flag==1]
    Predict -> Correct [order 2] : [flag==1]
    Predict -> AutoSlowDown [order 1] : [i>=0.6*N && flag!=1]
    AutoSlowDown -> Correct : [flag==1]
    Correct -> Correct [order 2] : [flag==1]
        | {i=0; iSD=0; diSD=1}
  data: targD input double size=nDOF+1; flag input uint32; comD output double size=nDOF+1; comV output double size=nDOF+1; comA output double size=nDOF+1; state output uint32; i output double; N output uint32 =256; nDOF parameter uint32 =1; di local double; diSD local double; iSD local double; targLocal local double size=nDOF+1; dtCon parameter double; dtSim parameter double; dtInt parameter double; dofID local uint32; vDOF local double; vDOFmax local double
